simulink model "rate_transition"  (R2018b)
settings: Solver=FixedStepDiscrete  StartTime=0.0  StopTime=10.0  FixedStep=0.1  RelTol=1e-3
settings Model: Creator=marwan  LastModifiedBy=marwan

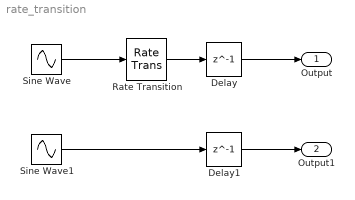
== system rate_transition ==
  Delay : Delay  DelayLength=1  SampleTime=1
  Delay1 : Delay  DelayLength=1  SampleTime=1
  Rate Transition : RateTransition
  Sine Wave : Sin  SampleTime=0.2
  Sine Wave1 : Sin  SampleTime=0.2
  Output : Outport
  Output1 : Outport  Port=2
  wires:
  Sine Wave/1 -> Rate Transition/1
  Delay/1 -> Output/1
  Delay1/1 -> Output1/1
  Rate Transition/1 -> Delay/1
  Sine Wave1/1 -> Delay1/1
